simulink model "Cascade_Controller_SIM"  (R2025b)
settings: Solver=FixedStepAuto  StartTime=0.0  StopTime=tspan  FixedStep=dt_sim  RelTol=rel_tol  AbsTol=abs_tol
undefined symbols (not defined in the file): mission_file
settings Model: Creator=koryh  LastModifiedBy=cyclone

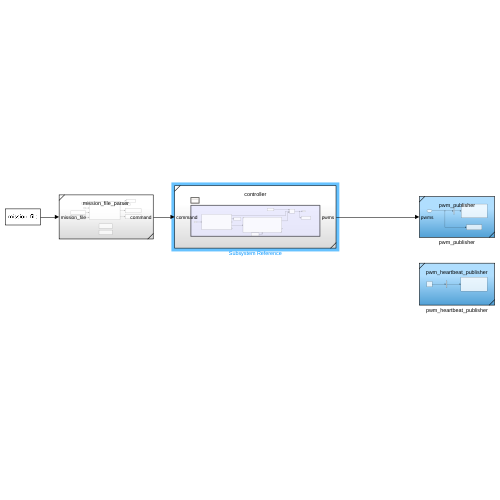
[thumbnail: Simulink's stored preview of the top-level diagram]
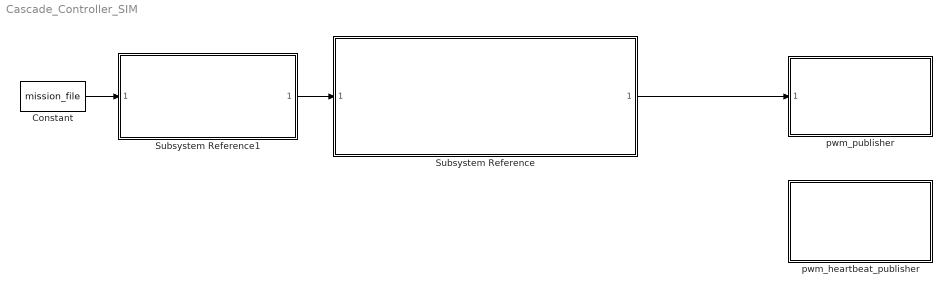
== system Cascade_Controller_SIM ==
  Constant : Constant  Value=mission_file
  Subsystem Reference : Subsystem  ReferencedSubsystem=controller
  Subsystem Reference1 : Subsystem  ReferencedSubsystem=mission_file_parser
  pwm_heartbeat_publisher : Subsystem  ReferencedSubsystem=pwm_heartbeat_publisher
  pwm_publisher : Subsystem  ReferencedSubsystem=pwm_publisher
  wires:
  Subsystem Reference/1 -> pwm_publisher/1
  Subsystem Reference1/1 -> Subsystem Reference/1
  Constant/1 -> Subsystem Reference1/1
